simulink model "six_pulse"  (R2024b)
settings: Solver=VariableStepAuto  StartTime=0  StopTime=tfinal  MaxStep=1e-6  RelTol=1e-3
InitFcn:
  | R_snubber = 24;
  | C_snubber = 2.2e-6;
  | R1_snubber = 0.001;
  | K = 1;
  | A = 141;
  | L = 6E-6;
undefined symbols (not defined in the file): dt_sim
libraries: spsSeriesRLCBranchLib x22, spsCurrentMeasurementLib x6, spsThyristorLib x6, spsACVoltageSourceLib x3, spsVoltageMeasurementLib x3, spsThreePhaseVIMeasurementLib x1, spsControlledCurrentSourceLib x1, spsGroundLib x1, spspowerguiLib x1
settings Model: Creator=Zongze.Wang  LastModifiedBy=XixiLab
settings SolverCC: ZeroCrossAlgorithm=Adaptive
settings DataIOCC: ExternalInput=[t0, u0']  InitialState=y0'  SaveFormat=Array  ReturnWorkspaceOutputs=off
settings DebuggingCC: IgnoredZcDiagnostic=none  UnconnectedInputMsg=warning  UnconnectedOutputMsg=warning  UnconnectedLineMsg=warning
settings ModelReferenceCC: EnableRefExpFcnMdlSchedulingChecks=on
settings RTWCC: GPUComputeCapability=3.5  DLArmComputeVersion=19.05

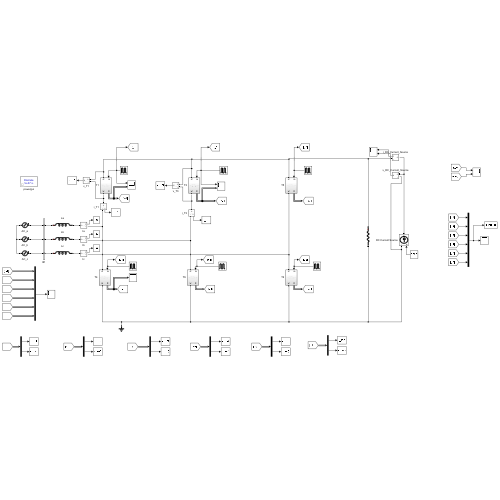
[thumbnail: Simulink's stored preview of the top-level diagram]
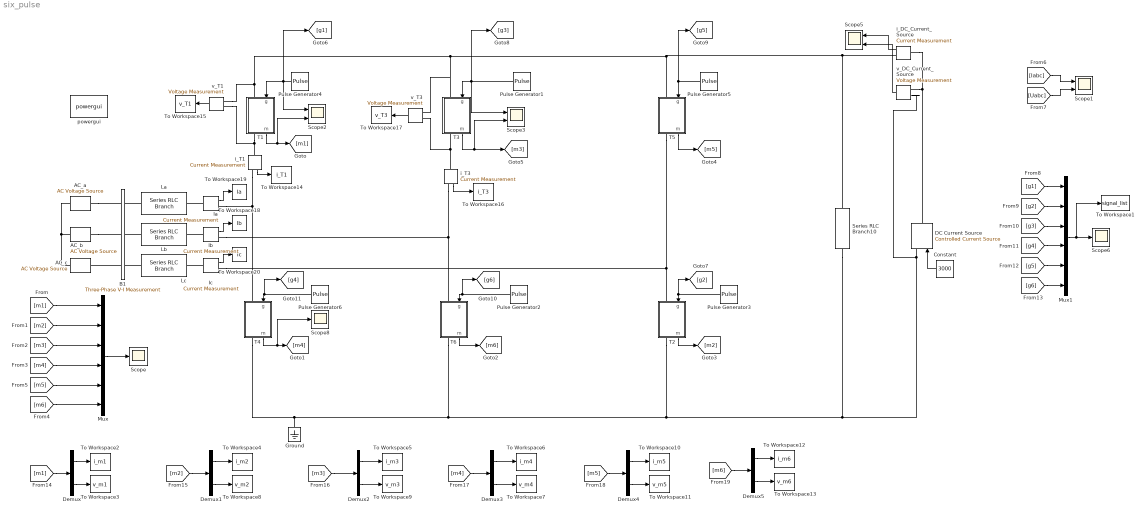
== system six_pulse ==
  AC_a : spsACVoltageSourceLib/AC Voltage Source  Amplitude=2074  Phase=21  Frequency=50  SampleTime=0  Measurements=None  BusType=swing  Pref=10e3  Qref=0  Qmin=-inf  Qmax=+inf
  AC_b : spsACVoltageSourceLib/AC Voltage Source  Amplitude=2074  Phase=261  Frequency=50  SampleTime=0  Measurements=None  BusType=swing  Pref=10e3  Qref=0  Qmin=-inf  Qmax=+inf
  AC_c : spsACVoltageSourceLib/AC Voltage Source  Amplitude=2074  Phase=141  Frequency=50  SampleTime=0  Measurements=None  BusType=swing  Pref=10e3  Qref=0  Qmin=-inf  Qmax=+inf
  B1 : spsThreePhaseVIMeasurementLib/Three-Phase V-I Measurement  VoltageMeasurement=phase-to-phase  SetLabelV=on  LabelV=Uabc  Vpu=off  VpuLL=off  CurrentMeasurement=yes  SetLabelI=on  LabelI=Iabc  Ipu=off  Pbase=200e6  Vbase=230e3  OutputType=Magnitude  PhasorSimulation=off  PSBequivalent=0
  Constant : Constant  Value=3000
  DC Current Source : spsControlledCurrentSourceLib/Controlled Current Source  Initialize=on  Source_Type=DC  Amplitude=2000  Phase=0  Frequency=0  Measurements=None
  Demux{,1..5} (6 alike) : Demux  Outputs=2
  Ground : spsGroundLib/Ground  LConnTagsString=a
  Ia : spsCurrentMeasurementLib/Current Measurement  PhasorSimulation=off  OutputType=Complex  PSBequivalent=0
  Ib : spsCurrentMeasurementLib/Current Measurement  PhasorSimulation=off  OutputType=Complex  PSBequivalent=0
  Ic : spsCurrentMeasurementLib/Current Measurement  PhasorSimulation=off  OutputType=Complex  PSBequivalent=0
  La : spsSeriesRLCBranchLib/Series RLC Branch  LConnTagsString=__new0  RConnTagsString=__new0  BranchType=L  Resistance=1  Inductance=312.5e-6*K  SetiL0=off  InitialCurrent=0  Capacitance=1e-6  Setx0=off  InitialVoltage=0  Measurements=None
  Lb : spsSeriesRLCBranchLib/Series RLC Branch  LConnTagsString=__new0  RConnTagsString=__new0  BranchType=L  Resistance=1  Inductance=312.5e-6*K  SetiL0=on  InitialCurrent=3000  Capacitance=1e-6  Setx0=off  InitialVoltage=0  Measurements=None
  Lc : spsSeriesRLCBranchLib/Series RLC Branch  LConnTagsString=__new0  RConnTagsString=__new0  BranchType=L  Resistance=1  Inductance=312.50e-6*K  SetiL0=on  InitialCurrent=-3000  Capacitance=1e-6  Setx0=off  InitialVoltage=0  Measurements=None
  Mux : Mux  Inputs=6
  Mux1 : Mux  Inputs=6
  Pulse Generator1 : DiscretePulseGenerator  PulseType=Time based  Amplitude=5  Period=0.02  PulseWidth=25  PhaseDelay=0.02/6+0.02/12
  Pulse Generator2 : DiscretePulseGenerator  PulseType=Time based  Amplitude=5  Period=0.02  PulseWidth=25  PhaseDelay=0.02/3*2+0.02/12
  Pulse Generator3 : DiscretePulseGenerator  PulseType=Time based  Amplitude=5  Period=0.02  PulseWidth=25  PhaseDelay=0.02/12
  Pulse Generator4 : DiscretePulseGenerator  PulseType=Time based  Amplitude=5  Period=0.02  PulseWidth=25  PhaseDelay=0.1/6+0.02/12
  Pulse Generator5 : DiscretePulseGenerator  PulseType=Time based  Amplitude=5  Period=0.02  PulseWidth=25  PhaseDelay=0.02/2+0.02/12
  Pulse Generator6 : DiscretePulseGenerator  PulseType=Time based  Amplitude=5  Period=0.02  PulseWidth=25  PhaseDelay=0.02/3+0.02/12
  Scope : Scope
  Scope{1..3,5} (4 alike) : Scope  NumInputPorts=2
  Scope6 : Scope
  Scope8 : Scope
  Series RLC Branch10 : spsSeriesRLCBranchLib/Series RLC Branch  LConnTagsString=__new0  RConnTagsString=__new0  BranchType=R  Resistance=1e7  Inductance=100e-6*K  SetiL0=on  InitialCurrent=0  Capacitance=1e-6  Setx0=off  InitialVoltage=0  Measurements=None
  T1 : Subsystem
      settings: PortSchema="{\"entries\":[{\"content\":{\"sides\":[{\"content\":{\"connectorIds\":[\"LConn1\",\"In1\"]},\"type\":\"ConnectorPlacement.EquallySpacedRectSide\",\"uuid\":\"aa3356c8-d33f-4a71-92cb-cede0495ab59\"},{\"content\":{\"connectorIds\":[\"RConn1\",\"Out1\"],\"side\":\"RIGHT\"},\"type\":\"ConnectorPlacement.EquallySpacedRectSide\",\"uuid\":\"8f7e1067-b902-4bf5-86c3-adc8f618f197\"},{\"content\":{\"connectorIds\":[],\"side\":\"TOP\"},\"type\":\"ConnectorPlacement.EquallySpacedRectSide\",\"uuid\":\"ca0505a9-d8b2-494f-8ec2-d8ddc53e3dda\"}]},\"type\":\"ConnectorPlacement.EquallySpacedConnector\",\"uuid\":\"bd09ced5-b41f-4ada-9ac3-69e98af1b82c\"}],\"packageUris\":[\"http://schema.mathworks.com/mf0/Connector/R2020b\"],\"version\":\"1.0\"}"
  T2 : Subsystem
      settings: PortSchema="{\"entries\":[{\"content\":{\"sides\":[{\"content\":{\"connectorIds\":[\"LConn1\",\"In1\"]},\"type\":\"ConnectorPlacement.EquallySpacedRectSide\",\"uuid\":\"aa3356c8-d33f-4a71-92cb-cede0495ab59\"},{\"content\":{\"connectorIds\":[\"RConn1\",\"Out1\"],\"side\":\"RIGHT\"},\"type\":\"ConnectorPlacement.EquallySpacedRectSide\",\"uuid\":\"8f7e1067-b902-4bf5-86c3-adc8f618f197\"},{\"content\":{\"connectorIds\":[],\"side\":\"TOP\"},\"type\":\"ConnectorPlacement.EquallySpacedRectSide\",\"uuid\":\"ca0505a9-d8b2-494f-8ec2-d8ddc53e3dda\"}]},\"type\":\"ConnectorPlacement.EquallySpacedConnector\",\"uuid\":\"bd09ced5-b41f-4ada-9ac3-69e98af1b82c\"}],\"packageUris\":[\"http://schema.mathworks.com/mf0/Connector/R2020b\"],\"version\":\"1.0\"}"
  T3 : Subsystem
      settings: PortSchema="{\"entries\":[{\"content\":{\"sides\":[{\"content\":{\"connectorIds\":[\"LConn1\",\"In1\"]},\"type\":\"ConnectorPlacement.EquallySpacedRectSide\",\"uuid\":\"aa3356c8-d33f-4a71-92cb-cede0495ab59\"},{\"content\":{\"connectorIds\":[\"RConn1\",\"Out1\"],\"side\":\"RIGHT\"},\"type\":\"ConnectorPlacement.EquallySpacedRectSide\",\"uuid\":\"8f7e1067-b902-4bf5-86c3-adc8f618f197\"},{\"content\":{\"connectorIds\":[],\"side\":\"TOP\"},\"type\":\"ConnectorPlacement.EquallySpacedRectSide\",\"uuid\":\"ca0505a9-d8b2-494f-8ec2-d8ddc53e3dda\"}]},\"type\":\"ConnectorPlacement.EquallySpacedConnector\",\"uuid\":\"bd09ced5-b41f-4ada-9ac3-69e98af1b82c\"}],\"packageUris\":[\"http://schema.mathworks.com/mf0/Connector/R2020b\"],\"version\":\"1.0\"}"
  T4 : Subsystem
      settings: PortSchema="{\"entries\":[{\"content\":{\"sides\":[{\"content\":{\"connectorIds\":[\"LConn1\",\"In1\"]},\"type\":\"ConnectorPlacement.EquallySpacedRectSide\",\"uuid\":\"aa3356c8-d33f-4a71-92cb-cede0495ab59\"},{\"content\":{\"connectorIds\":[\"RConn1\",\"Out1\"],\"side\":\"RIGHT\"},\"type\":\"ConnectorPlacement.EquallySpacedRectSide\",\"uuid\":\"8f7e1067-b902-4bf5-86c3-adc8f618f197\"},{\"content\":{\"connectorIds\":[],\"side\":\"TOP\"},\"type\":\"ConnectorPlacement.EquallySpacedRectSide\",\"uuid\":\"ca0505a9-d8b2-494f-8ec2-d8ddc53e3dda\"}]},\"type\":\"ConnectorPlacement.EquallySpacedConnector\",\"uuid\":\"bd09ced5-b41f-4ada-9ac3-69e98af1b82c\"}],\"packageUris\":[\"http://schema.mathworks.com/mf0/Connector/R2020b\"],\"version\":\"1.0\"}"
  T5 : Subsystem
      settings: PortSchema="{\"entries\":[{\"content\":{\"sides\":[{\"content\":{\"connectorIds\":[\"LConn1\",\"In1\"]},\"type\":\"ConnectorPlacement.EquallySpacedRectSide\",\"uuid\":\"aa3356c8-d33f-4a71-92cb-cede0495ab59\"},{\"content\":{\"connectorIds\":[\"RConn1\",\"Out1\"],\"side\":\"RIGHT\"},\"type\":\"ConnectorPlacement.EquallySpacedRectSide\",\"uuid\":\"8f7e1067-b902-4bf5-86c3-adc8f618f197\"},{\"content\":{\"connectorIds\":[],\"side\":\"TOP\"},\"type\":\"ConnectorPlacement.EquallySpacedRectSide\",\"uuid\":\"ca0505a9-d8b2-494f-8ec2-d8ddc53e3dda\"}]},\"type\":\"ConnectorPlacement.EquallySpacedConnector\",\"uuid\":\"bd09ced5-b41f-4ada-9ac3-69e98af1b82c\"}],\"packageUris\":[\"http://schema.mathworks.com/mf0/Connector/R2020b\"],\"version\":\"1.0\"}"
  T6 : Subsystem
      settings: PortSchema="{\"entries\":[{\"content\":{\"sides\":[{\"content\":{\"connectorIds\":[\"LConn1\",\"In1\"]},\"type\":\"ConnectorPlacement.EquallySpacedRectSide\",\"uuid\":\"aa3356c8-d33f-4a71-92cb-cede0495ab59\"},{\"content\":{\"connectorIds\":[\"RConn1\",\"Out1\"],\"side\":\"RIGHT\"},\"type\":\"ConnectorPlacement.EquallySpacedRectSide\",\"uuid\":\"8f7e1067-b902-4bf5-86c3-adc8f618f197\"},{\"content\":{\"connectorIds\":[],\"side\":\"TOP\"},\"type\":\"ConnectorPlacement.EquallySpacedRectSide\",\"uuid\":\"ca0505a9-d8b2-494f-8ec2-d8ddc53e3dda\"}]},\"type\":\"ConnectorPlacement.EquallySpacedConnector\",\"uuid\":\"bd09ced5-b41f-4ada-9ac3-69e98af1b82c\"}],\"packageUris\":[\"http://schema.mathworks.com/mf0/Connector/R2020b\"],\"version\":\"1.0\"}"
  To Workspace1 : ToWorkspace  VariableName=signal_list  SampleTime=-1
      settings: Save2DSignal=2-D array (concatenate along first dimension)
  To Workspace10 : ToWorkspace  VariableName=i_m5  SampleTime=-1
      settings: Save2DSignal=2-D array (concatenate along first dimension)
  To Workspace11 : ToWorkspace  VariableName=v_m5  SampleTime=-1
      settings: Save2DSignal=2-D array (concatenate along first dimension)
  To Workspace12 : ToWorkspace  VariableName=i_m6  SampleTime=-1
      settings: Save2DSignal=2-D array (concatenate along first dimension)
  To Workspace13 : ToWorkspace  VariableName=v_m6  SampleTime=-1
      settings: Save2DSignal=2-D array (concatenate along first dimension)
  To Workspace14 : ToWorkspace  VariableName=i_T1  SampleTime=-1
      settings: Save2DSignal=2-D array (concatenate along first dimension)
  To Workspace15 : ToWorkspace  VariableName=v_T1  SampleTime=-1
      settings: Save2DSignal=2-D array (concatenate along first dimension)
  To Workspace16 : ToWorkspace  VariableName=i_T3  SampleTime=-1
      settings: Save2DSignal=2-D array (concatenate along first dimension)
  To Workspace17 : ToWorkspace  VariableName=v_T3  SampleTime=-1
      settings: Save2DSignal=2-D array (concatenate along first dimension)
  To Workspace18 : ToWorkspace  VariableName=Ib  SampleTime=-1
      settings: Save2DSignal=2-D array (concatenate along first dimension)
  To Workspace19 : ToWorkspace  VariableName=Ia  SampleTime=-1
      settings: Save2DSignal=2-D array (concatenate along first dimension)
  To Workspace2 : ToWorkspace  VariableName=i_m1  SampleTime=-1
      settings: Save2DSignal=2-D array (concatenate along first dimension)
  To Workspace20 : ToWorkspace  VariableName=Ic  SampleTime=-1
      settings: Save2DSignal=2-D array (concatenate along first dimension)
  To Workspace3 : ToWorkspace  VariableName=v_m1  SampleTime=-1
      settings: Save2DSignal=2-D array (concatenate along first dimension)
  To Workspace4 : ToWorkspace  VariableName=i_m2  SampleTime=-1
      settings: Save2DSignal=2-D array (concatenate along first dimension)
  To Workspace5 : ToWorkspace  VariableName=i_m3  SampleTime=-1
      settings: Save2DSignal=2-D array (concatenate along first dimension)
  To Workspace6 : ToWorkspace  VariableName=i_m4  SampleTime=-1
      settings: Save2DSignal=2-D array (concatenate along first dimension)
  To Workspace7 : ToWorkspace  VariableName=v_m4  SampleTime=-1
      settings: Save2DSignal=2-D array (concatenate along first dimension)
  To Workspace8 : ToWorkspace  VariableName=v_m2  SampleTime=-1
      settings: Save2DSignal=2-D array (concatenate along first dimension)
  To Workspace9 : ToWorkspace  VariableName=v_m3  SampleTime=-1
      settings: Save2DSignal=2-D array (concatenate along first dimension)
  i_DC_Current_Source : spsCurrentMeasurementLib/Current Measurement  PhasorSimulation=off  OutputType=Complex  PSBequivalent=0
  i_T1 : spsCurrentMeasurementLib/Current Measurement  PhasorSimulation=off  OutputType=Complex  PSBequivalent=0
  i_T3 : spsCurrentMeasurementLib/Current Measurement  PhasorSimulation=off  OutputType=Complex  PSBequivalent=0
  powergui : spspowerguiLib/powergui  Priority=1  SimulationMode=Discrete  SampleTime=dt_sim  frequency=60  Iterations=50  frequencyindice=50  Pbase=100e6  ErrMax=1e-4  UnitsV=kV  UnitsW=MW  buscounter=0  FunctionMessages=off  echomessages=off  EnableUseOfTLC=off  CurrentSourceSwitches=on  DisableSnubberDevices=off  DisableRonSwitches=off  DisableVfSwitches=off  DisplayEquations=off  AutomaticDiscreteSolvers=off  SolverType=Tustin/Backward Euler (TBE)  Interpol=off  ExternalGateDelay=off  methode=off  Ts=10  x0status=blocks  SPID=off  SwTol=0  HookPort=off  NonlinearTolerance=0  nMaxIteration=15  ContinueOnMaxIteration=off  RestoreLinks=warning  ResistiveCurrentMeasurement=off  Frange=[0:2:500]  Ylog=off  Xlog=on  ShowGrid=off  save=off  variable=ZData  structure=0  ZoomFFT=off  StartTime=0.0  cycles=1  DisplayStyle=1  fundamental=60  FreqAxis=off  MaxFrequency=1000  frequencyindicesteady=1  RmsSteady=1  display=off
  v_DC_Current_Source : spsVoltageMeasurementLib/Voltage Measurement  PhasorSimulation=off  OutputType=Complex  PSBequivalent=0
  v_T1 : spsVoltageMeasurementLib/Voltage Measurement  PhasorSimulation=off  OutputType=Complex  PSBequivalent=0
  v_T3 : spsVoltageMeasurementLib/Voltage Measurement  PhasorSimulation=off  OutputType=Complex  PSBequivalent=0
  wires:
  Constant/1 -> DC Current Source/1
  Pulse Generator3/1 -> [g2], T2/1(g)
  T1/1(m) -> Scope2/2, [m1]
  [Uabc] -> Scope1/2
  [Iabc] -> Scope1/1
  [m2] -> Mux/2
  [m6] -> Mux/6
  Mux/1 -> Scope/1
  [m1] -> Mux/1
  T6/1(m) -> [m6]
  T4/1(m) -> Scope8/1, [m4]
  [m4] -> Mux/4
  T2/1(m) -> [m2]
  Pulse Generator1/1 -> [g3], Scope3/1, T3/1(g)
  [m3] -> Mux/3
  Pulse Generator2/1 -> [g6], T6/1(g)
  Pulse Generator4/1 -> [g1], Scope2/1, T1/1(g)
  Pulse Generator6/1 -> [g4], T4/1(g)
  [m5] -> Mux/5
  T5/1(m) -> [m5]
  T3/1(m) -> [m3], Scope3/2
  Pulse Generator5/1 -> T5/1(g), [g5]
  v_DC_Current_Source/1 -> Scope5/2
  i_DC_Current_Source/1 -> Scope5/1
  [g1] -> Mux1/1
  [g2] -> Mux1/2
  [g3] -> Mux1/3
  [g4] -> Mux1/4
  [g5] -> Mux1/5
  [g6] -> Mux1/6
  Mux1/1 -> To Workspace1/1, Scope6/1
  [m1] -> Demux/1
  Demux/1 -> To Workspace2/1
  Demux/2 -> To Workspace3/1
  [m2] -> Demux1/1
  Demux1/1 -> To Workspace4/1
  Demux1/2 -> To Workspace8/1
  [m3] -> Demux2/1
  Demux2/1 -> To Workspace5/1
  Demux2/2 -> To Workspace9/1
  [m4] -> Demux3/1
  Demux3/1 -> To Workspace6/1
  Demux3/2 -> To Workspace7/1
  [m5] -> Demux4/1
  Demux4/1 -> To Workspace10/1
  Demux4/2 -> To Workspace11/1
  [m6] -> Demux5/1
  Demux5/1 -> To Workspace12/1
  Demux5/2 -> To Workspace13/1
  i_T1/1 -> To Workspace14/1
  v_T1/1 -> To Workspace15/1
  i_T3/1 -> To Workspace16/1
  v_T3/1 -> To Workspace17/1
  Ib/1 -> To Workspace18/1
  Ia/1 -> To Workspace19/1
  Ic/1 -> To Workspace20/1
  connections:
  AC_b/LConn1 -- AC_c/LConn1 -- AC_a/LConn1
  i_T1/RConn1 -- Ia/RConn1 -- T4/LConn1
  AC_a/RConn1 -- B1/LConn1
  i_DC_Current_Source/LConn1 -- v_DC_Current_Source/LConn1 -- DC Current Source/RConn1
  AC_b/RConn1 -- B1/LConn2
  B1/LConn3 -- AC_c/RConn1
  v_DC_Current_Source/LConn2 -- DC Current Source/LConn1 -- Series RLC Branch10/RConn1 -- T2/RConn1 -- T6/RConn1 -- T4/RConn1 -- Ground/LConn1
  i_DC_Current_Source/RConn1 -- Series RLC Branch10/LConn1 -- T5/LConn1 -- v_T3/LConn1 -- T3/LConn1 -- v_T1/LConn1 -- T1/LConn1
  T5/RConn1 -- Ic/RConn1 -- T2/LConn1
  i_T3/RConn1 -- Ib/RConn1 -- T6/LConn1
  La/LConn1 -- B1/RConn1
  Lb/LConn1 -- B1/RConn2
  Lc/LConn1 -- B1/RConn3
  T1/RConn1 -- v_T1/LConn2 -- i_T1/LConn1
  i_T3/LConn1 -- T3/RConn1 -- v_T3/LConn2
  Ib/LConn1 -- Lb/RConn1
  Ia/LConn1 -- La/RConn1
  Ic/LConn1 -- Lc/RConn1

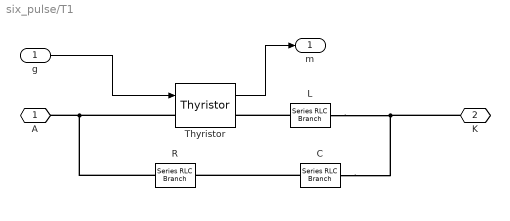
== system six_pulse/T1 ==
  g : Inport
  C : spsSeriesRLCBranchLib/Series RLC Branch  LConnTagsString=__new0  RConnTagsString=__new0  BranchType=C  Resistance=36  Inductance=1.9e-3  SetiL0=off  InitialCurrent=0  Capacitance=C_snubber*K  Setx0=off  InitialVoltage=0  Measurements=None
  L : spsSeriesRLCBranchLib/Series RLC Branch  LConnTagsString=__new0  RConnTagsString=__new0  BranchType=L  Resistance=36  Inductance=5e-6  SetiL0=off  InitialCurrent=0  Capacitance=C_snubber*K  Setx0=off  InitialVoltage=0  Measurements=None
  R : spsSeriesRLCBranchLib/Series RLC Branch  LConnTagsString=__new0  RConnTagsString=__new0  BranchType=R  Resistance=R_snubber*K  Inductance=1.9e-3  SetiL0=off  InitialCurrent=0  Capacitance=1e-6  Setx0=off  InitialVoltage=0  Measurements=None
  Thyristor : spsThyristorLib/Thyristor  Ron=0.001  Lon=0  Vf=0.8  IC=0  Rs=1e5  Cs=inf  Measurements=on
  A : PMIOPort  Side=Left
  K : PMIOPort  Port=2  Side=Right
  m : Outport
  wires:
  g/1 -> Thyristor/1
  Thyristor/1 -> m/1
  connections:
  K/RConn1 -- L/RConn1 -- C/RConn1
  Thyristor/LConn1 -- R/LConn1 -- A/RConn1
  C/LConn1 -- R/RConn1
  L/LConn1 -- Thyristor/RConn1

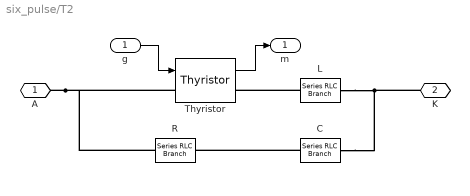
== system six_pulse/T2 ==
  g : Inport
  C : spsSeriesRLCBranchLib/Series RLC Branch  LConnTagsString=__new0  RConnTagsString=__new0  BranchType=C  Resistance=36  Inductance=1.9e-3  SetiL0=off  InitialCurrent=0  Capacitance=C_snubber*K  Setx0=off  InitialVoltage=0  Measurements=None
  L : spsSeriesRLCBranchLib/Series RLC Branch  LConnTagsString=__new0  RConnTagsString=__new0  BranchType=L  Resistance=36  Inductance=5e-6  SetiL0=off  InitialCurrent=0  Capacitance=C_snubber*K  Setx0=off  InitialVoltage=0  Measurements=None
  R : spsSeriesRLCBranchLib/Series RLC Branch  LConnTagsString=__new0  RConnTagsString=__new0  BranchType=R  Resistance=R_snubber*K  Inductance=1.9e-3  SetiL0=off  InitialCurrent=0  Capacitance=1e-6  Setx0=off  InitialVoltage=0  Measurements=None
  Thyristor : spsThyristorLib/Thyristor  Ron=0.001  Lon=0  Vf=0.8  IC=0  Rs=1e5  Cs=inf  Measurements=on
  A : PMIOPort  Side=Left
  K : PMIOPort  Port=2  Side=Right
  m : Outport
  wires:
  g/1 -> Thyristor/1
  Thyristor/1 -> m/1
  connections:
  C/RConn1 -- K/RConn1 -- L/RConn1
  A/RConn1 -- Thyristor/LConn1 -- R/LConn1
  C/LConn1 -- R/RConn1
  L/LConn1 -- Thyristor/RConn1

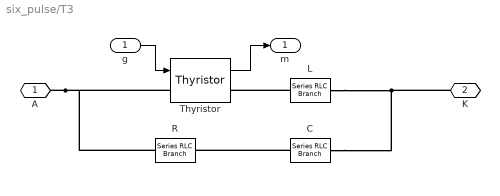
== system six_pulse/T3 ==
  g : Inport
  C : spsSeriesRLCBranchLib/Series RLC Branch  LConnTagsString=__new0  RConnTagsString=__new0  BranchType=C  Resistance=36  Inductance=1.9e-3  SetiL0=off  InitialCurrent=0  Capacitance=C_snubber*K  Setx0=off  InitialVoltage=0  Measurements=None
  L : spsSeriesRLCBranchLib/Series RLC Branch  LConnTagsString=__new0  RConnTagsString=__new0  BranchType=L  Resistance=36  Inductance=5e-6  SetiL0=off  InitialCurrent=0  Capacitance=C_snubber*K  Setx0=off  InitialVoltage=0  Measurements=None
  R : spsSeriesRLCBranchLib/Series RLC Branch  LConnTagsString=__new0  RConnTagsString=__new0  BranchType=R  Resistance=R_snubber*K  Inductance=1.9e-3  SetiL0=off  InitialCurrent=0  Capacitance=1e-6  Setx0=off  InitialVoltage=0  Measurements=None
  Thyristor : spsThyristorLib/Thyristor  Ron=0.001  Lon=0  Vf=0.8  IC=0  Rs=1e5  Cs=inf  Measurements=on
  A : PMIOPort  Side=Left
  K : PMIOPort  Port=2  Side=Right
  m : Outport
  wires:
  g/1 -> Thyristor/1
  Thyristor/1 -> m/1
  connections:
  C/RConn1 -- K/RConn1 -- L/RConn1
  A/RConn1 -- Thyristor/LConn1 -- R/LConn1
  C/LConn1 -- R/RConn1
  L/LConn1 -- Thyristor/RConn1

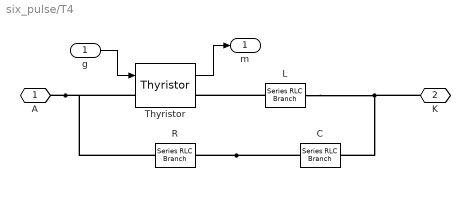
== system six_pulse/T4 ==
  g : Inport
  C : spsSeriesRLCBranchLib/Series RLC Branch  LConnTagsString=__new0  RConnTagsString=__new0  BranchType=C  Resistance=36  Inductance=1.9e-3  SetiL0=off  InitialCurrent=0  Capacitance=C_snubber*K  Setx0=off  InitialVoltage=0  Measurements=None
  L : spsSeriesRLCBranchLib/Series RLC Branch  LConnTagsString=__new0  RConnTagsString=__new0  BranchType=L  Resistance=36  Inductance=5e-6  SetiL0=off  InitialCurrent=0  Capacitance=C_snubber*K  Setx0=off  InitialVoltage=0  Measurements=None
  R : spsSeriesRLCBranchLib/Series RLC Branch  LConnTagsString=__new0  RConnTagsString=__new0  BranchType=R  Resistance=R_snubber*K  Inductance=1.9e-3  SetiL0=off  InitialCurrent=0  Capacitance=1e-6  Setx0=off  InitialVoltage=0  Measurements=None
  Thyristor : spsThyristorLib/Thyristor  Ron=0.001  Lon=0  Vf=0.8  IC=0  Rs=1e5  Cs=inf  Measurements=on
  A : PMIOPort  Side=Left
  K : PMIOPort  Port=2  Side=Right
  m : Outport
  wires:
  g/1 -> Thyristor/1
  Thyristor/1 -> m/1
  connections:
  K/RConn1 -- L/RConn1 -- C/RConn1
  A/RConn1 -- Thyristor/LConn1 -- R/LConn1
  R/RConn1 -- C/LConn1
  L/LConn1 -- Thyristor/RConn1

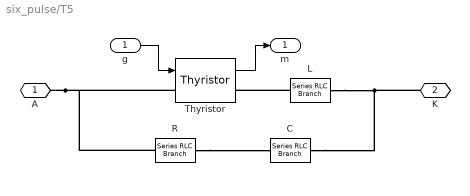
== system six_pulse/T5 ==
  g : Inport
  C : spsSeriesRLCBranchLib/Series RLC Branch  LConnTagsString=__new0  RConnTagsString=__new0  BranchType=C  Resistance=36  Inductance=1.9e-3  SetiL0=off  InitialCurrent=0  Capacitance=C_snubber*K  Setx0=off  InitialVoltage=0  Measurements=None
  L : spsSeriesRLCBranchLib/Series RLC Branch  LConnTagsString=__new0  RConnTagsString=__new0  BranchType=L  Resistance=36  Inductance=5e-6  SetiL0=off  InitialCurrent=0  Capacitance=C_snubber*K  Setx0=off  InitialVoltage=0  Measurements=None
  R : spsSeriesRLCBranchLib/Series RLC Branch  LConnTagsString=__new0  RConnTagsString=__new0  BranchType=R  Resistance=R_snubber*K  Inductance=1.9e-3  SetiL0=off  InitialCurrent=0  Capacitance=1e-6  Setx0=off  InitialVoltage=0  Measurements=None
  Thyristor : spsThyristorLib/Thyristor  Ron=0.001  Lon=0  Vf=0.8  IC=0  Rs=1e5  Cs=inf  Measurements=on
  A : PMIOPort  Side=Left
  K : PMIOPort  Port=2  Side=Right
  m : Outport
  wires:
  g/1 -> Thyristor/1
  Thyristor/1 -> m/1
  connections:
  C/RConn1 -- K/RConn1 -- L/RConn1
  A/RConn1 -- Thyristor/LConn1 -- R/LConn1
  R/RConn1 -- C/LConn1
  L/LConn1 -- Thyristor/RConn1

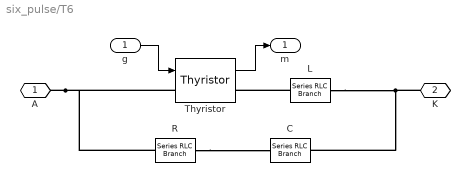
== system six_pulse/T6 ==
  g : Inport
  C : spsSeriesRLCBranchLib/Series RLC Branch  LConnTagsString=__new0  RConnTagsString=__new0  BranchType=C  Resistance=36  Inductance=1.9e-3  SetiL0=off  InitialCurrent=0  Capacitance=C_snubber*K  Setx0=off  InitialVoltage=0  Measurements=None
  L : spsSeriesRLCBranchLib/Series RLC Branch  LConnTagsString=__new0  RConnTagsString=__new0  BranchType=L  Resistance=36  Inductance=5e-6  SetiL0=off  InitialCurrent=0  Capacitance=C_snubber*K  Setx0=off  InitialVoltage=0  Measurements=None
  R : spsSeriesRLCBranchLib/Series RLC Branch  LConnTagsString=__new0  RConnTagsString=__new0  BranchType=R  Resistance=R_snubber*K  Inductance=1.9e-3  SetiL0=off  InitialCurrent=0  Capacitance=1e-6  Setx0=off  InitialVoltage=0  Measurements=None
  Thyristor : spsThyristorLib/Thyristor  Ron=0.001  Lon=0  Vf=0.8  IC=0  Rs=1e5  Cs=inf  Measurements=on
  A : PMIOPort  Side=Left
  K : PMIOPort  Port=2  Side=Right
  m : Outport
  wires:
  g/1 -> Thyristor/1
  Thyristor/1 -> m/1
  connections:
  K/RConn1 -- L/RConn1 -- C/RConn1
  A/RConn1 -- Thyristor/LConn1 -- R/LConn1
  R/RConn1 -- C/LConn1
  L/LConn1 -- Thyristor/RConn1
